simulink model "Pellet_softening_reactor"  (Simulink 8.5)
settings: Solver=ode23tb  SolverMode=SingleTasking  StartTime=0.0  StopTime=25*24*3600
undefined symbols (not defined in the file or in its folder): B, U, x0
settings Model: Creator=psross  LastModifiedBy=Martijn  ExtModeTrigMode=oneshot  ExtModeArmWhenConnect=off
settings DataIOCC: LimitDataPoints=off  SaveOutput=off  SaveTime=off  SignalLoggingName=sigsOut
settings OptimizationCC: BooleanDataType=off
settings DebuggingCC: SaveWithParameterizedLinksMsg=none  SignalResolutionControl=TryResolveAllWithWarning  MultiTaskDSMMsg=warning  MultiTaskCondExecSysMsg=none  FcnCallInpInsideContextMsg=UseLocalSettings  StrictBusMsg=None
settings HardwareCC: TargetUnknown=on

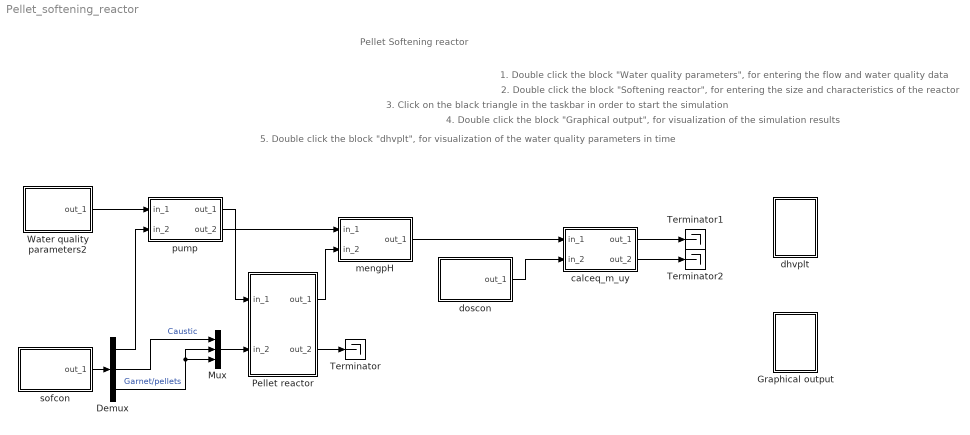
== system Pellet_softening_reactor ==
  note: Pellet Softening reactor
  note: 3. Click on the black triangle in the taskbar in order to start the simulation
  note: 4. Double click the block "Graphical output", for visualization of the simulation results
  note: 1. Double click the block "Water quality parameters", for entering the flow and water quality data
  note: 2. Double click the block "Softening reactor", for entering the size and characteristics of the reactor
  note: 5. Double click the block "dhvplt", for visualization of the water quality parameters in time
  Demux : Demux  Outputs=3
  Graphical output : Subsystem
      settings: OpenFcn=pels25_g
      mask Display:
      | plot(0,0,100,100,[80,20,20],[20,20,80],[80,69,60,52,45,39,33,28,24,20],[65,65,64,61,57,52,45,37,30,20])
      | disp('');
      | text(100,100,'pels25', 'horizontalAlignment', 'right', 'verticalAlignment', 'top');
  Mux : Mux  Inputs=3
  Pellet reactor : Subsystem  Description=pelsof 25
      mask init:
      | filenaam='./StimelaData/pelsof_p.mat';
      | 
      | [Pn,Fn,Fext]=Fileprop(filenaam);
      | 
      | errstr = st_UniqName(filenaam,'filenaam=''','SubSystem','OpenFcn');
      | if errstr, error([errstr 'The filename "' filenaam '" is already in use. Choose a different filename.']), end
      | 
      | P = pels25_p(filenaam);
      | [B,x0,U]=pels25_i(filenaam);
      settings: OpenFcn=|
      | filenaam='./StimelaData/pelsof_p.mat';
      | st_ParameterInput('init',gcb,filenaam,'pels25');
      mask Display:
      | image(imread('pels25_f.jpg'))
      | plot(0,0,100,100)
      | disp('')
      | text(50,50,'pels25', 'horizontalAlignment', 'center', 'verticalAlignment', 'middle');
      | text(50,0,Fn, 'horizontalAlignment', 'center', 'verticalAlignment', 'base');
  Terminator : Terminator
  Terminator1 : Terminator
  Terminator2 : Terminator
  Water quality parameters2 : Subsystem  Description=The water flow and the water quality data must be filled out in the 'Water quality parameters' block. Each project must start with a 'Water quality parameters' block.
      mask init:
      | filenaam='./StimelaData/invoerruw.mat';
      | 
      | [Pn,Fn,Fext]=Fileprop(filenaam);
      | 
      | errstr = st_UniqName(filenaam,'filenaam=''','SubSystem','OpenFcn');
      | if errstr, error([errstr 'The filename "' filenaam '" is already in use. Choose a different filename.']), end
      | 
      | P = invruw_p(filenaam);
      | [B,x0,U]=invruw_i(filenaam);
      settings: OpenFcn=|
      | filenaam='./StimelaData/invoerruw.mat';
      | st_ParameterInput('init',gcb,filenaam,'invruw');
      mask Display:
      | plot(0,0,100,100,[80 100],[ 50 50],[80 100],[ 55 55],[20 80 80 20 20],[10 10 90  90 10]);
      | disp('')
      | text(50,50,'invruw', 'horizontalAlignment', 'center', 'verticalAlignment', 'middle');
      | text(50,0,Fn, 'horizontalAlignment', 'center', 'verticalAlignment', 'base');
  calceq_m_uy : Subsystem  Description=calceq
      mask init:
      | filenaam='./StimelaData/calceq_p.mat';
      | 
      | [Pn,Fn,Fext]=Fileprop(filenaam);
      | 
      | errstr = st_UniqName(filenaam,'filenaam=''','SubSystem','OpenFcn');
      | if errstr, error([errstr 'The filename "' filenaam '" is already in use. Choose a different filename.']), end
      | 
      | P = calceq_p(filenaam);
      | [B,x0,U]=calceq_i(filenaam);
      settings: OpenFcn=|
      | filenaam='./StimelaData/calceq_p.mat';
      | st_ParameterInput('init',gcb,filenaam,'calceq');
      mask Display:
      | plot(0,0,100,100,[0 20],[80 80],[0 20],[85 85],[0 20],[20 20],[80 100],[80 80],[80 100],[85 85],[80 100],[ 20 20],[20 80 80 20 20],[10 10 90  90 10]);
      | text(50,50,'calceq', 'horizontalAlignment', 'center', 'verticalAlignment', 'middle');
      | text(0,0,filenaam, 'horizontalAlignment', 'left', 'verticalAlignment', 'bottom');
      | disp('')
      | text(50,50,'calceq', 'horizontalAlignment', 'center', 'verticalAlignment', 'middle');
      | text(50,0,Fn, 'horizontalAlignment', 'center', 'verticalAlignment', 'base');
  dhvplt : Subsystem
      settings: OpenFcn=plotStimela2
      mask Display:
      | plot(0,0,100,100,[80,20,20],[20,20,80],[80,69,60,52,45,39,33,28,24,20],[65,65,64,61,57,52,45,37,30,20])
      | disp('');
      | text(100,100,'Stimela', 'horizontalAlignment', 'right', 'verticalAlignment', 'top');
  doscon : Subsystem  Description=doscon
      mask init:
      | filenaam='./StimelaData/doscon_p.mat';
      | 
      | [Pn,Fn,Fext]=Fileprop(filenaam);
      | 
      | errstr = st_UniqName(filenaam,'filenaam=''','SubSystem','OpenFcn');
      | if errstr, error([errstr 'The filename "' filenaam '" is already in use. Choose a different filename.']), end
      | 
      | P = doscon_p(filenaam);
      | [B,x0,U]=doscon_i(filenaam);
      settings: OpenFcn=|
      | filenaam='./StimelaData/doscon_p.mat';
      | st_ParameterInput('init',gcb,filenaam,'doscon');
      mask Display:
      | plot(0,0,100,100,[80 100],[ 50 50],[80 100],[ 55 55],[20 80 80 20 20],[10 10 90  90 10]);
      | disp('')
      | text(50,50,'doscon', 'horizontalAlignment', 'center', 'verticalAlignment', 'middle');
      | text(50,0,Fn, 'horizontalAlignment', 'center', 'verticalAlignment', 'base');
  mengpH : Subsystem  Description=mengpH
      mask init:
      | filenaam='./StimelaData/mengpH_p.mat';
      | 
      | [Pn,Fn,Fext]=Fileprop(filenaam);
      | 
      | errstr = st_UniqName(filenaam,'filenaam=''','SubSystem','OpenFcn');
      | if errstr, error([errstr 'The filename "' filenaam '" is already in use. Choose a different filename.']), end
      | 
      | P = mengpH_p(filenaam);
      | [B,x0,U]=mengpH_i(filenaam);
      | V = st_Varia;
      settings: OpenFcn=|
      | filenaam='./StimelaData/mengpH_p.mat';
      | st_ParameterInput('init',gcb,filenaam,'mengpH');
      mask Display:
      | plot(0,0,100,100,[0 20],[85 85],[0 20],[80 80],[0 20],[20 20],[0 20],[15 15],[80 100],[ 50 50],[80 100],[ 55 55],[20 80 80 20 20],[10 10 90  90 10]);
      | disp('')
      | text(50,50,'mengpH', 'horizontalAlignment', 'center', 'verticalAlignment', 'middle');
      | text(50,0,Fn, 'horizontalAlignment', 'center', 'verticalAlignment', 'base');
  pump : Subsystem  Description=pomper
      mask init:
      | filenaam='./StimelaData/pomper_p.mat';
      | 
      | [Pn,Fn,Fext]=Fileprop(filenaam);
      | 
      | errstr = st_UniqName(filenaam,'filenaam=''','SubSystem','OpenFcn');
      | if errstr, error([errstr 'The filename "' filenaam '" is already in use. Choose a different filename.']), end
      | 
      | P = pomper_p(filenaam);
      | [B,x0,U]=pomper_i(filenaam);
      settings: OpenFcn=|
      | filenaam='./StimelaData/pomper_p.mat';
      | st_ParameterInput('init',gcb,filenaam,'pomper');
      mask Display:
      | plot(0,0,100,100,[0 20],[80 80],[0 20],[85 85],[0 20],[20 20],[80 100],[80 80],[80 100],[85 85],[80 100],[ 20 20],[80 100],[ 15 15],[20 80 80 20 20],[10 10 90  90 10]);
      | disp('')
      | text(50,50,'pomper', 'horizontalAlignment', 'center', 'verticalAlignment', 'middle');
      | text(50,0,Fn, 'horizontalAlignment', 'center', 'verticalAlignment', 'base');
  sofcon : Subsystem  Description=sofcon
      mask init:
      | filenaam='./StimelaData/sofcon_p.mat';
      | 
      | [Pn,Fn,Fext]=Fileprop(filenaam);
      | 
      | errstr = st_UniqName(filenaam,'filenaam=''','SubSystem','OpenFcn');
      | if errstr, error([errstr 'The filename "' filenaam '" is already in use. Choose a different filename.']), end
      | 
      | P = sofcon_p(filenaam);
      | [B,x0,U]=sofcon_i(filenaam);
      settings: OpenFcn=|
      | filenaam='./StimelaData/sofcon_p.mat';
      | st_ParameterInput('init',gcb,filenaam,'sofcon');
      mask Display:
      | plot(0,0,100,100,[80 100],[ 50 50],[80 100],[ 55 55],[20 80 80 20 20],[10 10 90  90 10]);
      | disp('')
      | text(50,50,'sofcon', 'horizontalAlignment', 'center', 'verticalAlignment', 'middle');
      | text(50,0,Fn, 'horizontalAlignment', 'center', 'verticalAlignment', 'base');
  wires:
  pump/2(out_2) -> mengpH/1(in_1)
  pump/1(out_1) -> Pellet reactor/1(in_1)
  Water quality parameters2/1(out_1) -> pump/1(in_1)
  Pellet reactor/1(out_1) -> mengpH/2(in_2)
  sofcon/1(out_1) -> Demux/1
  Demux/1 -> pump/2(in_2)
  Pellet reactor/2(out_2) -> Terminator/1
  doscon/1(out_1) -> calceq_m_uy/2(in_2)
  mengpH/1(out_1) -> calceq_m_uy/1(in_1)
  calceq_m_uy/1(out_1) -> Terminator1/1
  calceq_m_uy/2(out_2) -> Terminator2/1
  Demux/2 -> Mux/1  "Caustic"
  Demux/3 -> Mux/2, Mux/3  "Garnet/pellets"
  Mux/1 -> Pellet reactor/2(in_2)

== system Pellet_softening_reactor/Graphical output ==
  note: plotten

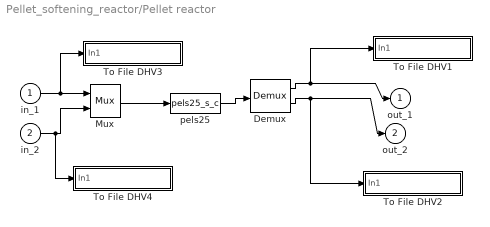
== system Pellet_softening_reactor/Pellet reactor ==
  in_1 : Inport
  in_2 : Inport  Port=2
  Demux : Demux  Outputs=[U.Number B.Measurements]
  Mux : Mux  Inputs=[U.Number B.Setpoints]
  To File DHV1 : Subsystem  mask(To File DHV){naam=[filenaam(1:length(filenaam)-4) '_out.sti']}
      mask prompts: naam "Naam van bestand"
      mask init:
      | set_param([gcb '/To File'],'Filename',naam);
      mask Display: disp(naam)
  To File DHV2 : Subsystem  mask(To File DHV){naam=[filenaam(1:length(filenaam)-4) '_EM.sti']}
      mask prompts: naam "Naam van bestand"
      mask init:
      | set_param([gcb '/To File'],'Filename',naam);
      mask Display: disp(naam)
  To File DHV3 : Subsystem  mask(To File DHV){naam=[filenaam(1:length(filenaam)-4) '_in.sti']}
      mask prompts: naam "Naam van bestand"
      mask init:
      | set_param([gcb '/To File'],'Filename',naam);
      mask Display: disp(naam)
  To File DHV4 : Subsystem  mask(To File DHV){naam=[filenaam(1:length(filenaam)-4) '_ES.sti']}
      mask prompts: naam "Naam van bestand"
      mask init:
      | set_param([gcb '/To File'],'Filename',naam);
      mask Display: disp(naam)
  pels25 : S-Function  FunctionName=pels25_s_c  Parameters=B,x0,U,P
  out_1 : Outport  InitialOutput=0
  out_2 : Outport  Port=2  InitialOutput=0
  wires:
  Demux/2 -> out_2/1, To File DHV2/1(In1)
  Demux/1 -> out_1/1, To File DHV1/1(In1)
  pels25/1 -> Demux/1
  in_1/1 -> Mux/1, To File DHV3/1(In1)
  Mux/1 -> pels25/1
  in_2/1 -> Mux/2, To File DHV4/1(In1)

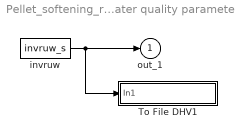
== system Pellet_softening_reactor/Water quality parameters2 ==
  To File DHV1 : Subsystem  mask(To File DHV){naam=[filenaam(1:length(filenaam)-4) '_out.sti']}
      mask prompts: naam "Naam van bestand"
      mask init:
      | set_param([gcb '/To File'],'Filename',naam);
      mask Display: disp(naam)
  invruw : S-Function  FunctionName=invruw_s  Parameters=B,x0,U,P
  out_1 : Outport  InitialOutput=0
  wires:
  invruw/1 -> out_1/1, To File DHV1/1(In1)

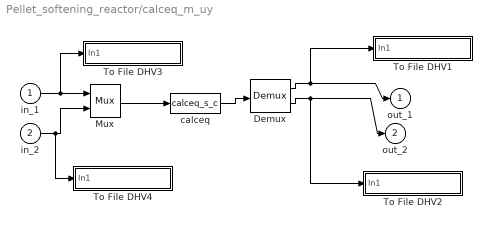
== system Pellet_softening_reactor/calceq_m_uy ==
  in_1 : Inport
  in_2 : Inport  Port=2
  Demux : Demux  Outputs=[U.Number B.Measurements]
  Mux : Mux  Inputs=[U.Number B.Setpoints]
  To File DHV1 : Subsystem  mask(To File DHV){naam=[filenaam(1:length(filenaam)-4) '_out.sti']}
      mask prompts: naam "Naam van bestand"
      mask init:
      | set_param([gcb '/To File'],'Filename',naam);
      mask Display: disp(naam)
  To File DHV2 : Subsystem  mask(To File DHV){naam=[filenaam(1:length(filenaam)-4) '_EM.sti']}
      mask prompts: naam "Naam van bestand"
      mask init:
      | set_param([gcb '/To File'],'Filename',naam);
      mask Display: disp(naam)
  To File DHV3 : Subsystem  mask(To File DHV){naam=[filenaam(1:length(filenaam)-4) '_in.sti']}
      mask prompts: naam "Naam van bestand"
      mask init:
      | set_param([gcb '/To File'],'Filename',naam);
      mask Display: disp(naam)
  To File DHV4 : Subsystem  mask(To File DHV){naam=[filenaam(1:length(filenaam)-4) '_ES.sti']}
      mask prompts: naam "Naam van bestand"
      mask init:
      | set_param([gcb '/To File'],'Filename',naam);
      mask Display: disp(naam)
  calceq : S-Function  FunctionName=calceq_s_c  Parameters=B,x0,U,P
  out_1 : Outport  InitialOutput=0
  out_2 : Outport  Port=2  InitialOutput=0
  wires:
  Demux/2 -> out_2/1, To File DHV2/1(In1)
  Demux/1 -> out_1/1, To File DHV1/1(In1)
  calceq/1 -> Demux/1
  in_1/1 -> Mux/1, To File DHV3/1(In1)
  Mux/1 -> calceq/1
  in_2/1 -> Mux/2, To File DHV4/1(In1)

== system Pellet_softening_reactor/dhvplt ==
  note: plotten

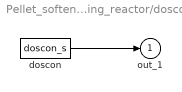
== system Pellet_softening_reactor/doscon ==
  doscon : S-Function  FunctionName=doscon_s  Parameters=B,x0,U,P
  out_1 : Outport  InitialOutput=0
  wires:
  doscon/1 -> out_1/1

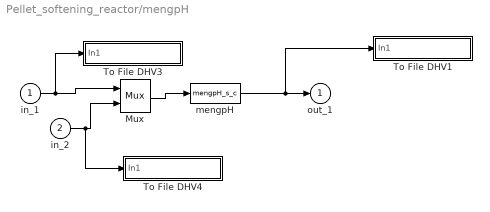
== system Pellet_softening_reactor/mengpH ==
  in_1 : Inport
  in_2 : Inport  Port=2
  Mux : Mux  Inputs=[U.Number B.Setpoints]
  To File DHV1 : Subsystem  mask(To File DHV){naam=[filenaam(1:length(filenaam)-4) '_out.sti']}
      mask prompts: naam "Naam van bestand"
      mask init:
      | set_param([gcb '/To File'],'Filename',naam);
      mask Display: disp(naam)
  To File DHV3 : Subsystem  mask(To File DHV){naam=[filenaam(1:length(filenaam)-4) '_in.sti']}
      mask prompts: naam "Naam van bestand"
      mask init:
      | set_param([gcb '/To File'],'Filename',naam);
      mask Display: disp(naam)
  To File DHV4 : Subsystem  mask(To File DHV){naam=[filenaam(1:length(filenaam)-4) '_ES.sti']}
      mask prompts: naam "Naam van bestand"
      mask init:
      | set_param([gcb '/To File'],'Filename',naam);
      mask Display: disp(naam)
  mengpH : S-Function  FunctionName=mengpH_s_c  Parameters=B,x0,U,P
  out_1 : Outport  InitialOutput=0
  wires:
  mengpH/1 -> out_1/1, To File DHV1/1(In1)
  Mux/1 -> mengpH/1
  in_1/1 -> Mux/1, To File DHV3/1(In1)
  in_2/1 -> Mux/2, To File DHV4/1(In1)

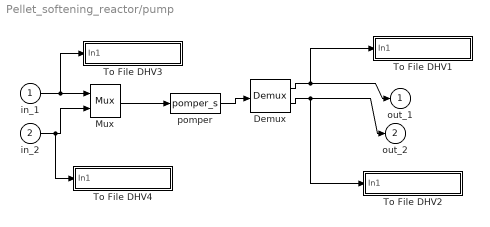
== system Pellet_softening_reactor/pump ==
  in_1 : Inport
  in_2 : Inport  Port=2
  Demux : Demux  Outputs=[U.Number B.Measurements]
  Mux : Mux  Inputs=[U.Number B.Setpoints]
  To File DHV1 : Subsystem  mask(To File DHV){naam=[filenaam(1:length(filenaam)-4) '_out.sti']}
      mask prompts: naam "Naam van bestand"
      mask init:
      | set_param([gcb '/To File'],'Filename',naam);
      mask Display: disp(naam)
  To File DHV2 : Subsystem  mask(To File DHV){naam=[filenaam(1:length(filenaam)-4) '_EM.sti']}
      mask prompts: naam "Naam van bestand"
      mask init:
      | set_param([gcb '/To File'],'Filename',naam);
      mask Display: disp(naam)
  To File DHV3 : Subsystem  mask(To File DHV){naam=[filenaam(1:length(filenaam)-4) '_in.sti']}
      mask prompts: naam "Naam van bestand"
      mask init:
      | set_param([gcb '/To File'],'Filename',naam);
      mask Display: disp(naam)
  To File DHV4 : Subsystem  mask(To File DHV){naam=[filenaam(1:length(filenaam)-4) '_ES.sti']}
      mask prompts: naam "Naam van bestand"
      mask init:
      | set_param([gcb '/To File'],'Filename',naam);
      mask Display: disp(naam)
  pomper : S-Function  FunctionName=pomper_s  Parameters=B,x0,U,P
  out_1 : Outport  InitialOutput=0
  out_2 : Outport  Port=2  InitialOutput=0
  wires:
  Demux/2 -> out_2/1, To File DHV2/1(In1)
  Demux/1 -> out_1/1, To File DHV1/1(In1)
  pomper/1 -> Demux/1
  in_1/1 -> Mux/1, To File DHV3/1(In1)
  Mux/1 -> pomper/1
  in_2/1 -> Mux/2, To File DHV4/1(In1)

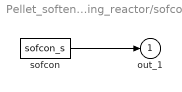
== system Pellet_softening_reactor/sofcon ==
  sofcon : S-Function  FunctionName=sofcon_s  Parameters=B,x0,U,P
  out_1 : Outport  InitialOutput=0
  wires:
  sofcon/1 -> out_1/1

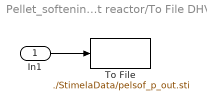
== system Pellet_softening_reactor/Pellet reactor/To File DHV1 ==
  In1 : Inport
  To File : ToFile  Filename=./StimelaData/pelsof_p_out.sti  MatrixName=pels25out
  wires:
  In1/1 -> To File/1

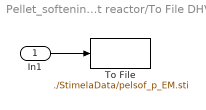
== system Pellet_softening_reactor/Pellet reactor/To File DHV2 ==
  In1 : Inport
  To File : ToFile  Filename=./StimelaData/pelsof_p_EM.sti  MatrixName=pels25EM
  wires:
  In1/1 -> To File/1

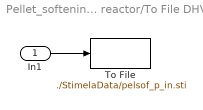
== system Pellet_softening_reactor/Pellet reactor/To File DHV3 ==
  In1 : Inport
  To File : ToFile  Filename=./StimelaData/pelsof_p_in.sti  MatrixName=pels25in
  wires:
  In1/1 -> To File/1

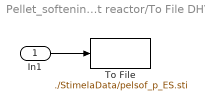
== system Pellet_softening_reactor/Pellet reactor/To File DHV4 ==
  In1 : Inport
  To File : ToFile  Filename=./StimelaData/pelsof_p_ES.sti  MatrixName=pels25ES
  wires:
  In1/1 -> To File/1

== system Pellet_softening_reactor/Water quality parameters2/To File DHV1 ==
  In1 : Inport
  To File : ToFile  Filename=./StimelaData/invoerruw_out.sti  MatrixName=invruwout
  wires:
  In1/1 -> To File/1

== system Pellet_softening_reactor/calceq_m_uy/To File DHV1 ==
  In1 : Inport
  To File : ToFile  Filename=./StimelaData/calceq_p_out.sti  MatrixName=calceqout
  wires:
  In1/1 -> To File/1

== system Pellet_softening_reactor/calceq_m_uy/To File DHV2 ==
  In1 : Inport
  To File : ToFile  Filename=./StimelaData/calceq_p_EM.sti  MatrixName=calceqEM
  wires:
  In1/1 -> To File/1

== system Pellet_softening_reactor/calceq_m_uy/To File DHV3 ==
  In1 : Inport
  To File : ToFile  Filename=./StimelaData/calceq_p_in.sti  MatrixName=calceqin
  wires:
  In1/1 -> To File/1

== system Pellet_softening_reactor/calceq_m_uy/To File DHV4 ==
  In1 : Inport
  To File : ToFile  Filename=./StimelaData/calceq_p_ES.sti  MatrixName=calceqES
  wires:
  In1/1 -> To File/1

== system Pellet_softening_reactor/mengpH/To File DHV1 ==
  In1 : Inport
  To File : ToFile  Filename=./StimelaData/mengpH_p_out.sti  MatrixName=mengpHout
  wires:
  In1/1 -> To File/1

== system Pellet_softening_reactor/mengpH/To File DHV3 ==
  In1 : Inport
  To File : ToFile  Filename=./StimelaData/mengpH_p_in.sti  MatrixName=mengpHin
  wires:
  In1/1 -> To File/1

== system Pellet_softening_reactor/mengpH/To File DHV4 ==
  In1 : Inport
  To File : ToFile  Filename=./StimelaData/mengpH_p_ES.sti  MatrixName=mengpHES
  wires:
  In1/1 -> To File/1

== system Pellet_softening_reactor/pump/To File DHV1 ==
  In1 : Inport
  To File : ToFile  Filename=./StimelaData/pomper_p_out.sti  MatrixName=pomperout
  wires:
  In1/1 -> To File/1

== system Pellet_softening_reactor/pump/To File DHV2 ==
  In1 : Inport
  To File : ToFile  Filename=./StimelaData/pomper_p_EM.sti  MatrixName=pomperEM
  wires:
  In1/1 -> To File/1

== system Pellet_softening_reactor/pump/To File DHV3 ==
  In1 : Inport
  To File : ToFile  Filename=./StimelaData/pomper_p_in.sti  MatrixName=pomperin
  wires:
  In1/1 -> To File/1

== system Pellet_softening_reactor/pump/To File DHV4 ==
  In1 : Inport
  To File : ToFile  Filename=./StimelaData/pomper_p_ES.sti  MatrixName=pomperES
  wires:
  In1/1 -> To File/1
